simulink model "Pend_Simscape_NN_Predictive"  (R2013a)
settings: Solver=ode45  StartTime=0.0  StopTime=5  RelTol=1e-3
values from neighbouring files (symbols this model uses):
  m = 0.2    [pendulum.m]    (also in pid.m; pid_control.m)
  s = rand(1,num_state)*initrange    [FastAHCCartPole.m]    (also in pendulum.m = tf('s'); pid.m = tf('s'); pid_control.m = tf('s'))
libraries: mblibv1 x13, neural x1
settings Model: Creator=Admin  LastModifiedBy=david78k
settings DataIOCC: SignalLoggingSaveFormat=ModelDataLogs
settings OptimizationCC: ExpressionDepthLimit=2147483647  InitFltsAndDblsToZero=on
settings DebuggingCC: AlgebraicLoopMsg=none  SolverPrmCheckMsg=none  FcnCallInpInsideContextMsg=UseLocalSettings  UnconnectedInputMsg=none  UnconnectedOutputMsg=none  UnconnectedLineMsg=none  StrictBusMsg=Warning
settings GRTTargetCC: CombineOutputUpdateFcns=off  GRTInterface=on
settings SimMechanicsCC: VisDuringSimulation=on

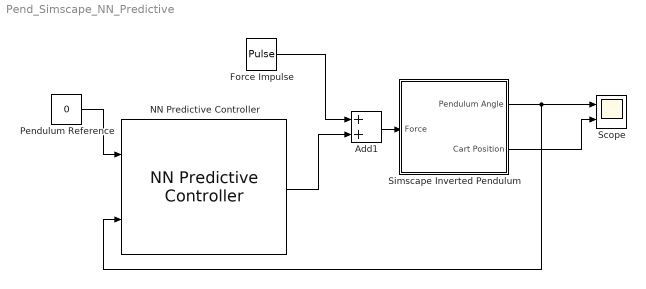
== system Pend_Simscape_NN_Predictive ==
  Add1 : Sum
  Force Impulse : DiscretePulseGenerator  PulseType=Time based  Amplitude=1000  Period=10  PulseWidth=0.01
  NN Predictive Controller : neural/Control Systems/NN Predictive Controller  epochs=200  minp=-4.1651718639737734  maxp=4.2831306231418793  mint=-3.1344028951578671  maxt=4.2831306231418793  Normalize=0  IW=[-0.51670339428008627 0.30216359067953968;0.063122064876303174 0.49648019761152751;-0.6011959254398701 0.51569845008084003;-0.33496484915941738 -0.21162981637168918;-1.1329233033622921 -0.79955533605292672;0.94071285967693519 0.41836714397439778;-0.8832550776227267 -0.76281244763460665]  LW1_2=[0.69782203805873777 -0.37077760385034442;0.34312334132666389 -0.89671763633998636;1.6999968221153436 -1.1019765395365144;-0.70848254525935916 0.23592009404776221;0.095950316508265771 -0.1506748459104448;0.39004078391021679 1.6160842305809311;0.45342855029825024 -0.028915641644308984]  LW2_1=[0.062190244781024681 -1.1043642367666291 1.377462760855878 -1.1466470424192063 -0.44306710436770214 -0.209459787239196 -0.032425765365737637]  B1=[3.4229281290107396;1.4885006445197408;-0.78178922136363049;0.15468020926256307;0.88460328618358486;-1.9180026772347927;2.6292228329429768]  B2=1.1926159034565735  max_i_int=20  min_i_int=5  limit_output=0  max_output=Inf  min_output=-Inf  Use_Previous_Weights=1  N2=7  Nu=2  Ts=0.2  rho=0.05  alpha=0.001  csrchfun=csrchbac  maxiter=2  S1=7  Ni=2  Nj=2  sim_file=Pend_Model_Simscape_oneout  trainfun=trainlm  Use_validation=1  Use_Testing=0  max_i=5  min_i=-5  sam_training=500
  Pendulum Reference : Constant  Value=0
  Scope : Scope  NumInputPorts=2
      settings: YMin=-5~-5  YMax=5~5
  Simscape Inverted Pendulum : Subsystem
  wires:
  Simscape Inverted Pendulum/1(Pendulum Angle) -> NN Predictive Controller/2, Scope/1
  Add1/1 -> Simscape Inverted Pendulum/1(Force)
  NN Predictive Controller/1 -> Add1/2
  Pendulum Reference/1 -> NN Predictive Controller/1
  Force Impulse/1 -> Add1/1
  Simscape Inverted Pendulum/2(Cart Position) -> Scope/2

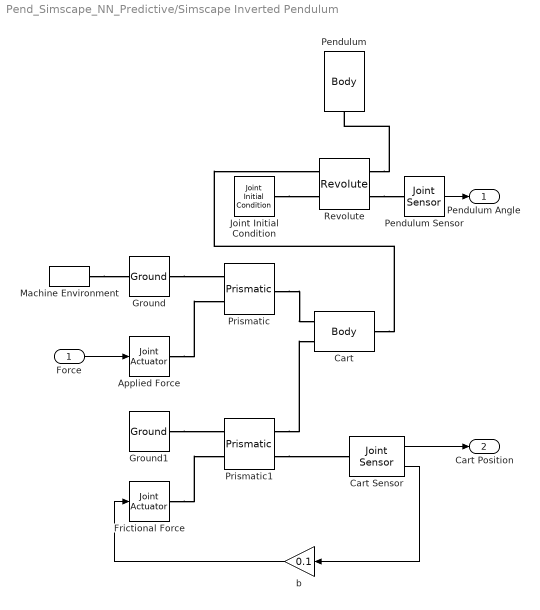
== system Pend_Simscape_NN_Predictive/Simscape Inverted Pendulum ==
  Force : Inport
  Applied Force : mblibv1/Sensors &  Actuators/Joint Actuator  UpdateFromCAD=off  PhysicalDomain=Mechanical  PortType=blob  ActuationStyle=Force  AngleUnits=deg  ArcVelocityUnits=deg/s  ArcAccelerationUnits=deg/s^2  CoordPositionUnits=m  VelocityUnits=m/s  AccelerationUnits=m/s^2  ForceUnits=N  TorqueUnits=N-m  ActiveIO=on  Width=1  DialogClass=MechanicalActuatorBlock  Primitive=P1  ReferenceFrame=Absolute (World)
  Cart : mblibv1/Bodies/Body  LConnTagsString=CS1|CS2  RConnTagsString=CS3  UpdateFromCAD=off  DialogClass=MechanicalBodyBlock  Mass=0.5  MassUnits=kg  InertiaUnits=kg*m^2  Inertia=eye(3)  Shape=Cylinder  ShapeDims=[1 1]  ShapeUnits=m  ShapeUse=false  Density=1  DensityUnits=kg/m^3  DensityUse=false  GraphicsMode=MACHINE_DEFAULT  BodyColorSelMode=MACHINE_DEFAULT  BodyColor=[1 0 0]  AttachedToCS=CG  CG=Left$CG$[0 0 0]$WORLD$WORLD$m$[0 0 0]$Euler X-Y-Z$deg$WORLD$false$none  WorkingFrames=Left$CS1$[-1 0 0]$CG$CG$m$[0 0 0]$Euler X-Y-Z$deg$WORLD$true$none#Left$CS2$[0 0 0]$CG$CG$m$[0 0 0]$Euler X-Y-Z$deg$WORLD$true$none#Right$CS3$[0 0.5 0]$CG$CG$m$[0 0 0]$Euler X-Y-Z$deg$WORLD$true$none#Right$CS4$[-1 0.5 0]$CG$CG$m$[0 0 0]$Euler X-Y-Z$deg$WORLD$false$none#Right$CS5$[-1 -0.5 0]$CG$CG$m$[0 0 0]$Euler X-Y-Z$deg$WORLD$false$none#Right$CS6$[1 -0.5 0]$CG$CG$m$[0 0 0]$Euler X-Y-Z$deg$WORLD$false$none#Right$CS7$[1 0.5 0]$CG$CG$m$[0 0 0]$Euler X-Y-Z$deg$WORLD$false$none  CGPos=[0 0 0]  CGRot=[0 0 0]  CS0Pos=[]  CS0Rot=[]  CS1Pos=[-1 0 0]  CS1Rot=[0 0 0]  CS2Pos=[0 0 0]  CS2Rot=[0 0 0]  CS3Pos=[0 0.5 0]  CS3Rot=[0 0 0]  CS4Pos=[-1 0.5 0]  CS4Rot=[0 0 0]  CS5Pos=[-1 -0.5 0]  CS5Rot=[0 0 0]  CS6Pos=[1 -0.5 0]  CS6Rot=[0 0 0]  CS7Pos=[1 0.5 0]  CS7Rot=[0 0 0]  CS8Pos=[]  CS8Rot=[]  CS9Pos=[]  CS9Rot=[]  CS10Pos=[]  CS10Rot=[]  CS11Pos=[]  CS11Rot=[]  CS12Pos=[]  CS12Rot=[]  CS13Pos=[]  CS13Rot=[]  CS14Pos=[]  CS14Rot=[]  CS15Pos=[]  CS15Rot=[]  CS16Pos=[]  CS16Rot=[]  CS17Pos=[]  CS17Rot=[]  CS18Pos=[]  CS18Rot=[]  CS19Pos=[]  CS19Rot=[]  CS20Pos=[]  CS20Rot=[]
  Cart Sensor : mblibv1/Sensors &  Actuators/Joint Sensor  UpdateFromCAD=off  PhysicalDomain=Mechanical  PortType=blob  Muxed=off  Pose=off  Angle=on  AngleUnits=deg  ArcVelocity=off  ArcVelocityUnits=deg/s  ArcAcceleration=off  ArcAccelerationUnits=deg/s^2  CoordPosition=on  CoordPositionUnits=m  Velocity=on  VelocityUnits=m/s  Acceleration=off  AccelerationUnits=m/s^2  Quaternion=on  QuaternionDT=off  QuaternionDDT=off  QuaternionUnits=off  OutputVector=[1]  ActiveIO=on  Width=2  DialogClass=MechanicalSensorBlock  Primitive=P1  Force=off  ForceUnits=N  Torque=off  TorqueUnits=N*m  ReferenceFrame=Absolute (World)  ReactionSensedSide=Base  ReactionReferenceFrame=Absolute (World)  ReactionForce=off  ReactionForceUnits=N  ReactionMoment=off  ReactionMomentUnits=N*m
  Frictional Force : mblibv1/Sensors &  Actuators/Joint Actuator  UpdateFromCAD=off  PhysicalDomain=Mechanical  PortType=blob  ActuationStyle=Force  AngleUnits=deg  ArcVelocityUnits=deg/s  ArcAccelerationUnits=deg/s^2  CoordPositionUnits=m  VelocityUnits=m/s  AccelerationUnits=m/s^2  ForceUnits=N  TorqueUnits=N*m  ActiveIO=on  Width=1  DialogClass=MechanicalActuatorBlock  Primitive=P1  ReferenceFrame=Absolute (World)
  Ground : mblibv1/Bodies/Ground  UpdateFromCAD=off  LeftPortType=env  RightPortType=workingframe  PhysicalDomain=Mechanical  DialogClass=GroundBlock  CoordPosition=[0 0 0]  CoordPositionUnits=m  StateVectorMgrId=-1  MachineId=[0 0]  ShowEnvPort=on
  Ground1 : mblibv1/Bodies/Ground  UpdateFromCAD=off  LeftPortType=env  RightPortType=workingframe  PhysicalDomain=Mechanical  DialogClass=GroundBlock  CoordPosition=[0 0 0]  CoordPositionUnits=m  StateVectorMgrId=-1  MachineId=[0 0]  ShowEnvPort=off
  Joint Initial Condition : mblibv1/Sensors &  Actuators/Joint Initial Condition  UpdateFromCAD=off  LeftPortType=blob  RightPortType=blob  PhysicalDomain=mechanical  DialogClass=InitialConditionBlock  InitialConditions=P1$false$0$m$deg$0$m/s$deg/s#P2$false$0$m$deg$0$m/s$deg/s#P3$false$0$m$deg$0$m/s$deg/s#R1$true$0$m$deg$0$m/s$deg/s#R2$false$0$m$deg$0$m/s$deg/s#R3$false$0$m$deg$0$m/s$deg/s#S$false$0$m$deg$0$m/s$deg/s  P1PIC=0  P1VIC=0  P2PIC=0  P2VIC=0  P3PIC=0  P3VIC=0  R1PIC=0  R1VIC=0  R2PIC=0  R2VIC=0  R3PIC=0  R3VIC=0  SPIC=0  SVIC=0
  Machine Environment : mblibv1/Bodies/Machine Environment  PortType=env  PhysicalDomain=Mechanical  DialogTemplateClass=MECH.MachineEnvironment  SyncWhenCopied=off  Gravity=[0 -9.81 0]  GravityUnits=m/s^2  GravityAsSignal=off  Dimensionality=Auto-detect  AnalysisType=Forward dynamics  LinearAssemblyTolerance=1e-3  LinearAssemblyToleranceUnits=m  AngularAssemblyTolerance=1e-3  AngularAssemblyToleranceUnits=rad  ConstraintSolverType=Stabilizing  ConstraintRelTolerance=1e-4  ConstraintAbsTolerance=1e-4  UseRobustSingularityHandling=off  RedundancyAnalysisToleranceType=Automatically select tolerance  RedundancyAnalysisTolerance=1e-14  StatePerturbationType=Fixed  PerturbationSize=1e-5  VisualizeMachine=on  BodyVisualizationType=Use model default body geometries  BodyColorSelMode=Use model default  DefaultBodyColor=[1 0 0]
  Pendulum : mblibv1/Bodies/Body  LConnTagsString=CS1  UpdateFromCAD=off  DialogClass=MechanicalBodyBlock  Mass=0.2  MassUnits=kg  InertiaUnits=kg*m^2  Inertia=0.006*eye(3)  Shape=Cylinder  ShapeDims=[1 1]  ShapeUnits=m  ShapeUse=false  Density=1  DensityUnits=kg/m^3  DensityUse=false  GraphicsMode=MACHINE_DEFAULT  BodyColorSelMode=COLORPALETTE  BodyColor=[0.078431 0.16863 0.54902]  AttachedToCS=CG  CG=Left$CG$[0 0.3 0]$CS1$CS1$m$[0 0 0]$Euler X-Y-Z$deg$WORLD$false$none  WorkingFrames=Left$CS1$[0 0 0]$Adjoining$Adjoining$m$[0 0 0]$Euler X-Y-Z$deg$WORLD$true$none#Right$CS2$[0.1 0 0]$CS1$CS1$m$[0 0 0]$Euler X-Y-Z$deg$WORLD$false$none#Right$CS3$[-0.1 0 0]$CS1$CS1$m$[0 0 0]$Euler X-Y-Z$deg$WORLD$false$none#Right$CS4$[-0.1 0.6 0]$CS1$CS1$m$[0 0 0]$Euler X-Y-Z$deg$WORLD$false$none#Right$CS5$[0.1 0.6 0]$CS1$CS1$m$[0 0 0]$Euler X-Y-Z$deg$WORLD$false$none  CGPos=[0 0.3 0]  CGRot=[0 0 0]  CS0Pos=[]  CS0Rot=[]  CS1Pos=[0 0 0]  CS1Rot=[0 0 0]  CS2Pos=[0.1 0 0]  CS2Rot=[0 0 0]  CS3Pos=[-0.1 0 0]  CS3Rot=[0 0 0]  CS4Pos=[-0.1 0.6 0]  CS4Rot=[0 0 0]  CS5Pos=[0.1 0.6 0]  CS5Rot=[0 0 0]  CS6Pos=[]  CS6Rot=[]  CS7Pos=[]  CS7Rot=[]  CS8Pos=[]  CS8Rot=[]  CS9Pos=[]  CS9Rot=[]  CS10Pos=[]  CS10Rot=[]  CS11Pos=[]  CS11Rot=[]  CS12Pos=[]  CS12Rot=[]  CS13Pos=[]  CS13Rot=[]  CS14Pos=[]  CS14Rot=[]  CS15Pos=[]  CS15Rot=[]  CS16Pos=[]  CS16Rot=[]  CS17Pos=[]  CS17Rot=[]  CS18Pos=[]  CS18Rot=[]  CS19Pos=[]  CS19Rot=[]  CS20Pos=[]  CS20Rot=[]
  Pendulum Sensor : mblibv1/Sensors &  Actuators/Joint Sensor  UpdateFromCAD=off  PhysicalDomain=Mechanical  PortType=blob  Muxed=on  Pose=off  Angle=on  AngleUnits=rad  ArcVelocity=off  ArcVelocityUnits=deg/s  ArcAcceleration=off  ArcAccelerationUnits=deg/s^2  CoordPosition=on  CoordPositionUnits=m  Velocity=off  VelocityUnits=m/s  Acceleration=off  AccelerationUnits=m/s^2  Quaternion=on  QuaternionDT=off  QuaternionDDT=off  QuaternionUnits=off  OutputVector=[1]  ActiveIO=on  Width=1  DialogClass=MechanicalSensorBlock  Primitive=R1  Force=off  ForceUnits=N  Torque=off  TorqueUnits=N*m  ReferenceFrame=Absolute (World)  ReactionSensedSide=Base  ReactionReferenceFrame=Absolute (World)  ReactionForce=off  ReactionForceUnits=N  ReactionMoment=off  ReactionMomentUnits=N*m
  Prismatic : mblibv1/Joints/Prismatic  LConnTagsString=__newl0|SA1  RConnTagsString=__newr0  UpdateFromCAD=off  NumSAPorts=1  CutJoint=off  MarkAsCut=off  Primitives=prismatic  PrimitiveProps=P1$World$[1 0 0]$prismatic  DialogClass=JointBlock  P1Axis=[1 0 0]
  Prismatic1 : mblibv1/Joints/Prismatic  LConnTagsString=__newl0|SA1  RConnTagsString=__newr0|SA1  UpdateFromCAD=off  NumSAPorts=2  CutJoint=off  MarkAsCut=off  Primitives=prismatic  PrimitiveProps=P1$World$[1 0 0]$prismatic  DialogClass=JointBlock  P1Axis=[1 0 0]
  Revolute : mblibv1/Joints/Revolute  LConnTagsString=__newl0|SA1  RConnTagsString=__newr0|SA1  UpdateFromCAD=off  NumSAPorts=2  CutJoint=off  MarkAsCut=off  Primitives=prismatic  PrimitiveProps=R1$World$[0 0 1]$revolute  DialogClass=JointBlock  R1Axis=[0 0 1]
  b : Gain  Gain=0.1
  Pendulum Angle : Outport
  Cart Position : Outport  Port=2
  wires:
  Cart Sensor/2 -> b/1
  b/1 -> Frictional Force/1
  Pendulum Sensor/1 -> Pendulum Angle/1
  Force/1 -> Applied Force/1
  Cart Sensor/1 -> Cart Position/1
  connections:
  Applied Force/RConn1 -- Prismatic/LConn2
  Prismatic/RConn1 -- Cart/LConn1
  Prismatic1/RConn1 -- Cart/LConn2
  Cart/RConn1 -- Revolute/LConn1
  Prismatic1/RConn2 -- Cart Sensor/LConn1
  Frictional Force/RConn1 -- Prismatic1/LConn2
  Machine Environment/RConn1 -- Ground/LConn1
  Ground/RConn1 -- Prismatic/LConn1
  Ground1/RConn1 -- Prismatic1/LConn1
  Joint Initial Condition/RConn1 -- Revolute/LConn2
  Revolute/RConn1 -- Pendulum/LConn1
  Revolute/RConn2 -- Pendulum Sensor/LConn1
